simulink model "obs"  (R2014b)
settings: Solver=ode3  StartTime=0.0  StopTime=1875  FixedStep=0.5e-3  RelTol=1e-3
values from neighbouring files (symbols this model uses):
  C1_array = [10000 10000 20775.14128 59367.58362 2271.12322 25499.34704 24626.77363 22758.69305 1470.76099 16269.06063 343.94923 166277.12244 ... (44 elements, 11x4)]    [ecmparams_vsc.mat]    (also in load_sim_data.m = [ecmparams(1:3,2)'; ecmparams(4:6,2)'; ecmparams(7:9,2)']; load_sim_data_v2.m = [ecmparams(1:3,2)'; ecmparams(4:6,2)'; ecmparams(7:9,2)'])
  C2_array = [5000 5000 3386.51997 1284.26954 733.57385 21.9068258 408.44714 1025.29527 23.88432 4732.43934 4.98786 7213.94612 ... (44 elements, 11x4)]    [ecmparams_vsc.mat]    (also in load_sim_data.m = [ecmparams(1:3,4)'; ecmparams(4:6,4)'; ecmparams(7:9,4)']; load_sim_data_v2.m = [ecmparams(1:3,4)'; ecmparams(4:6,4)'; ecmparams(7:9,4)'])
  drive_profile = [0.003069801 0.003247245 0.003020715 0.003053892 0.002820143 0.003317081 0.003158873 0.002919445 0.002956375 0.002698265 0.002861501 0.002770798 ... (18750 elements, 1x18750)]    [drive_profile_ftp.mat]    (also in workspace.mat = [0 0 0 0 0 0 0 0 0 0 0 0 ... (521 elements, 1x521)]; workspace_2rc.mat; workspace_comparison.mat)
  drive_profile_index = [1 2 3 4 5 6 7 8 9 10 11 12 ... (18750 elements, 1x18750)]    [drive_profile_ftp.mat]    (also in load_sim_data_v2.m = drive_profile_index - 1; workspace.mat = [0 0.115384615385 0.230769230769 0.346153846154 0.4615384615; workspace_2rc.mat; workspace_comparison.mat)
  exp_vterm = [3.629339 3.628863 3.628776 3.628435 3.628006 3.627681 3.627586 3.627112 3.626967 3.626491 3.626216 3.625935 ... (18750 elements, 18750x1)]    [exp_vterm.mat]    (also in workspace_2rc.mat; workspace_comparison.mat)
  exp_vterm_index = [1 2 3 4 5 6 7 8 9 10 11 12 ... (18750 elements, 18750x1)]    [exp_vterm.mat]    (also in load_sim_data_v2.m = exp_vterm_index - 1)
  initial_soc = interp1(voc_soc_lut, voc_soc_lut_index, initial_vterm)    [load_sim_data.m]    (also in load_sim_data_v2.m)
  initial_temp = 25    [load_sim_data.m]    (also in load_sim_data_v2.m)
  initial_voc = interp1(voc_soc_lut_index, voc_soc_lut, initial_soc)    [load_sim_data.m]    (also in load_sim_data_v2.m)
  Q_total = 236.8    [load_sim_data.m]    (also in load_sim_data_v2.m = 350; workspace.mat = 44; workspace_2rc.mat = 44; workspace_comparison.mat = 44)
  R1 = interp2(temp_array, voc_array, R1_array, initial_temp, initial_voc)    [load_sim_data.m]    (also in load_sim_data_v2.m; workspace.mat = 0.00033425; workspace_2rc.mat = 0.0001483; workspace_comparison.mat = 0.0001483)
  R1_array = [0.001 0.001 0.00171 0.00621 0.00621 0.00495 0.00657 0.00419 0.01404 0.0095 0.00356 0.01783 ... (44 elements, 11x4)]    [ecmparams_vsc.mat]    (also in load_sim_data.m = [ecmparams(1:3,3)'; ecmparams(4:6,3)'; ecmparams(7:9,3)']; load_sim_data_v2.m = [ecmparams(1:3,3)'; ecmparams(4:6,3)'; ecmparams(7:9,3)'])
  R2 = interp2(temp_array, voc_array, R2_array, initial_temp, initial_voc)    [load_sim_data.m]    (also in load_sim_data_v2.m; workspace.mat = 0.000915125; workspace_2rc.mat = 0.0001594; workspace_comparison.mat = 0.0001594)
  R2_array = [0.001 0.001 0.00067 0.01044 0.00794 0.01181 0.0098 0.00694 0.00323 0.00236 0.02009 0.00195 ... (44 elements, 11x4)]    [ecmparams_vsc.mat]    (also in load_sim_data.m = [ecmparams(1:3,5)'; ecmparams(4:6,5)'; ecmparams(7:9,5)']; load_sim_data_v2.m = [ecmparams(1:3,5)'; ecmparams(4:6,5)'; ecmparams(7:9,5)'])
  Ri = interp2(temp_array, voc_array, Ri_array, initial_temp, initial_voc)    [load_sim_data.m]    (also in load_sim_data_v2.m; workspace.mat = 0.000736040625; workspace_2rc.mat = 0.0007932; workspace_comparison.mat = 0.0007932)
  Ri_array = [0.001 0.001 0.00089 0.02157 0.01286 0.00303 0.0054 0.0079 0.00204 0.01221 0.00632 0.00315 ... (44 elements, 11x4)]    [ecmparams_vsc.mat]    (also in load_sim_data.m = [ecmparams(1:3,1)'; ecmparams(4:6,1)'; ecmparams(7:9,1)']; load_sim_data_v2.m = [ecmparams(1:3,1)'; ecmparams(4:6,1)'; ecmparams(7:9,1)'])
  T_est = 0.02    [load_sim_data.m]    (also in load_sim_data_v2.m)
  temp_array = [15 25 35]    [load_sim_data.m]    (also in load_sim_data_v2.m)
  voc_array = [3 3.6 4.2]    [load_sim_data.m]    (also in load_sim_data_v2.m)
  voc_soc_lut = [3.07420931 3.44278771 3.51037487 3.58546258 3.63776945 3.68066188 3.73931818 3.84140797 3.94332291 4.0535654 4.18301283]    [emf_curve_single.mat]    (also in workspace.mat = [2.9985 3.0047 3.1504 3.2397 3.3026 3.3438 3.3699 3.3878 3.4; workspace_2rc.mat = [2.9985 3.0047 3.1504 3.2397 3.3026 3.3438 3.3699 3.3878 3.4; workspace_comparison.mat = [2.9985 3.0047 3.1504 3.2397 3.3026 3.3438 3.3699 3.3878 3.4)
  voc_soc_lut_index = [0 10 20 30 40 50 60 70 80 90 100]    [emf_curve_single.mat]    (also in workspace.mat = [0 1.6393442623 3.27868852459 4.91803278689 6.55737704918 8.; workspace_2rc.mat = [0 1.6393442623 3.27868852459 4.91803278689 6.55737704918 8.; workspace_comparison.mat = [0 1.6393442623 3.27868852459 4.91803278689 6.55737704918 8.)
libraries: fl_lib x16, nesl_utility x10
settings Model: Creator=OTG00077  LastModifiedBy=OTG00077
settings DebuggingCC: MultiTaskRateTransMsg=warning

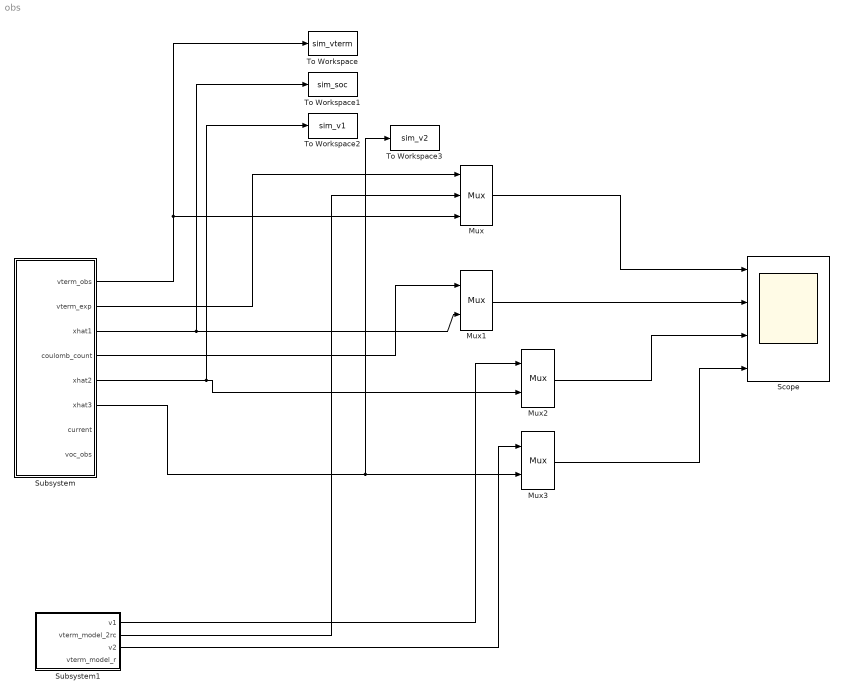
== system obs ==
  Mux : Mux  Inputs=3
  Mux1 : Mux  Inputs=2
  Mux2 : Mux  Inputs=2
  Mux3 : Mux  Inputs=2
  Scope : Scope  NumInputPorts=4
      settings: TimeRange=1875  YMin=3.458604651162791~0~-0.05~-0.05  YMax=3.741395348837209~40~0.009999999999999995~0.009999999999999995
  Subsystem : Subsystem
  Subsystem1 : Subsystem
  To Workspace : ToWorkspace  VariableName=sim_vterm  SampleTime=1
  To Workspace1 : ToWorkspace  VariableName=sim_soc  SampleTime=1
  To Workspace2 : ToWorkspace  VariableName=sim_v1  SampleTime=1
  To Workspace3 : ToWorkspace  VariableName=sim_v2  SampleTime=1
  wires:
  Subsystem/2(vterm_exp) -> Mux/1
  Subsystem1/2(vterm_model_2rc) -> Mux/2
  Subsystem/1(vterm_obs) -> To Workspace/1, Mux/3
  Subsystem/4(coulomb_count) -> Mux1/1
  Subsystem/3(xhat1) -> To Workspace1/1, Mux1/2
  Subsystem1/1(v1) -> Mux2/1
  Subsystem/5(xhat2) -> To Workspace2/1, Mux2/2
  Subsystem1/3(v2) -> Mux3/1
  Subsystem/6(xhat3) -> To Workspace3/1, Mux3/2
  Mux/1 -> Scope/1
  Mux1/1 -> Scope/2
  Mux2/1 -> Scope/3
  Mux3/1 -> Scope/4

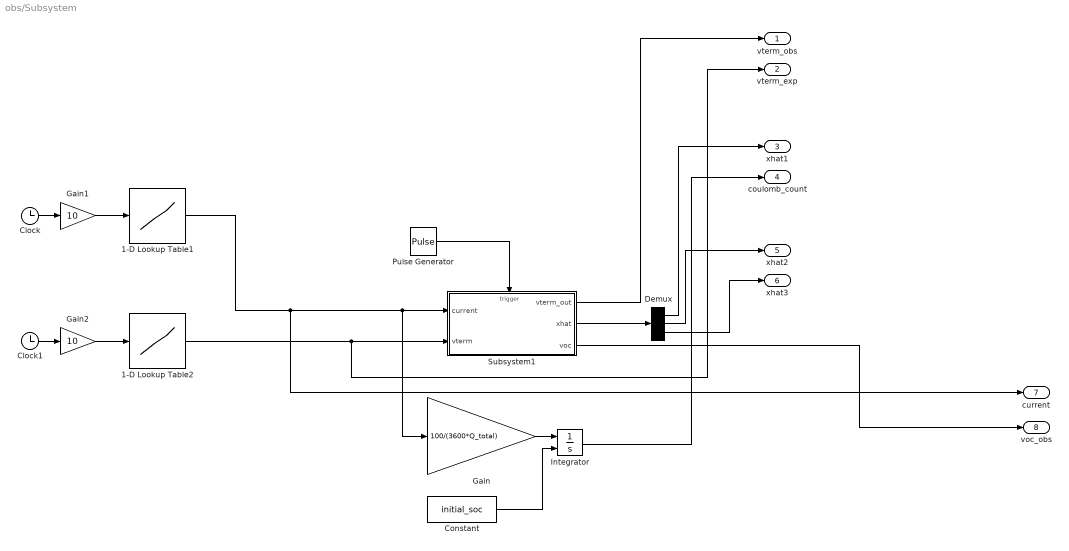
== system obs/Subsystem ==
  1-D Lookup Table1 : Lookup_n-D  NumberOfTableDimensions=1  BreakpointsForDimension1=drive_profile_index  Table=drive_profile  InternalRulePriority=Speed  RndMeth=Simplest  InputSameDT=on
  1-D Lookup Table2 : Lookup_n-D  NumberOfTableDimensions=1  BreakpointsForDimension1=exp_vterm_index  Table=exp_vterm  InternalRulePriority=Speed  RndMeth=Simplest  InputSameDT=on
  Clock : Clock
      settings: Decimation=100
  Clock1 : Clock
      settings: Decimation=100
  Constant : Constant  Value=initial_soc
  Demux : Demux  Outputs=3
  Gain : Gain  Gain=100/(3600*Q_total)
  Gain1 : Gain  Gain=10
  Gain2 : Gain  Gain=10
  Integrator : Integrator  InitialConditionSource=external  InitialCondition=initial_soc
  Pulse Generator : DiscretePulseGenerator  SampleTime=T_est/2
  Subsystem1 : Subsystem
  vterm_obs : Outport
  vterm_exp : Outport  Port=2
  xhat1 : Outport  Port=3
  coulomb_count : Outport  Port=4
  xhat2 : Outport  Port=5
  xhat3 : Outport  Port=6
  current : Outport  Port=7
  voc_obs : Outport  Port=8
  wires:
  Integrator/1 -> coulomb_count/1
  Gain/1 -> Integrator/1
  Pulse Generator/1 -> Subsystem1/Trigger
  1-D Lookup Table2/1 -> vterm_exp/1, Subsystem1/2(vterm)
  Subsystem1/2(xhat) -> Demux/1
  Clock1/1 -> Gain2/1
  Gain1/1 -> 1-D Lookup Table1/1
  Clock/1 -> Gain1/1
  1-D Lookup Table1/1 -> current/1, Gain/1, Subsystem1/1(current)
  Gain2/1 -> 1-D Lookup Table2/1
  Subsystem1/1(vterm_out) -> vterm_obs/1
  Demux/1 -> xhat1/1
  Constant/1 -> Integrator/2
  Demux/2 -> xhat2/1
  Demux/3 -> xhat3/1
  Subsystem1/3(voc) -> voc_obs/1

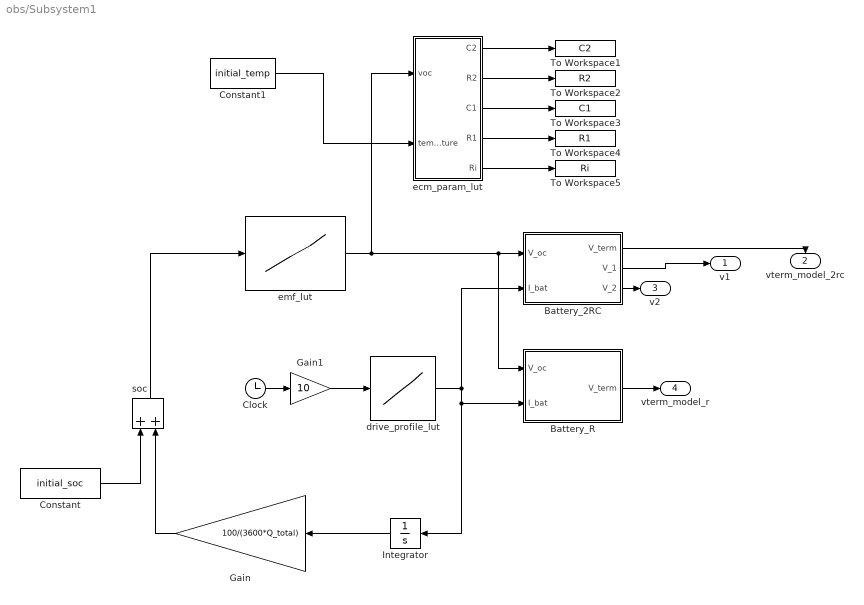
== system obs/Subsystem1 ==
  Battery_2RC : Subsystem
  Battery_R : Subsystem
  Clock : Clock
      settings: Decimation=100
  Constant : Constant  Value=initial_soc
  Constant1 : Constant  Value=initial_temp
  Gain : Gain  Gain=100/(3600*Q_total)
  Gain1 : Gain  Gain=10
  Integrator : Integrator
  To Workspace1 : ToWorkspace  VariableName=C2  SampleTime=-1
      settings: MaxDataPoints=1  Decimation=100
  To Workspace2 : ToWorkspace  VariableName=R2  SampleTime=-1
      settings: MaxDataPoints=1  Decimation=100
  To Workspace3 : ToWorkspace  VariableName=C1  SampleTime=-1
      settings: MaxDataPoints=1  Decimation=100
  To Workspace4 : ToWorkspace  VariableName=R1  SampleTime=-1
      settings: MaxDataPoints=1  Decimation=100
  To Workspace5 : ToWorkspace  VariableName=Ri  SampleTime=-1
      settings: MaxDataPoints=1  Decimation=100
  drive_profile_lut : Lookup_n-D  NumberOfTableDimensions=1  BreakpointsForDimension1=drive_profile_index  Table=drive_profile  InternalRulePriority=Speed  RndMeth=Simplest  InputSameDT=on
  "ecm_param_lut " : Subsystem
  emf_lut : Lookup_n-D  NumberOfTableDimensions=1  BreakpointsForDimension1=voc_soc_lut_index  Table=voc_soc_lut  InternalRulePriority=Speed  RndMeth=Simplest  InputSameDT=on
  soc : Sum
  v1 : Outport
  vterm_model_2rc : Outport  Port=2
  v2 : Outport  Port=3
  vterm_model_r : Outport  Port=4
  wires:
  "ecm_param_lut "/3(C1) -> To Workspace3/1
  "ecm_param_lut "/4(R1) -> To Workspace4/1
  Integrator/1 -> Gain/1
  Battery_2RC/2(V_1) -> v1/1
  Battery_2RC/3(V_2) -> v2/1
  Battery_2RC/1(V_term) -> vterm_model_2rc/1
  "ecm_param_lut "/5(Ri) -> To Workspace5/1
  Gain1/1 -> drive_profile_lut/1
  Battery_R/1(V_term) -> vterm_model_r/1
  "ecm_param_lut "/1(C2) -> To Workspace1/1
  "ecm_param_lut "/2(R2) -> To Workspace2/1
  drive_profile_lut/1 -> Battery_R/2(I_bat), Integrator/1, Battery_2RC/2(I_bat)
  Clock/1 -> Gain1/1
  emf_lut/1 -> "ecm_param_lut "/1(voc), Battery_R/1(V_oc), Battery_2RC/1(V_oc)
  Constant/1 -> soc/1
  Gain/1 -> soc/2
  soc/1 -> emf_lut/1
  Constant1/1 -> "ecm_param_lut "/2(temperature)

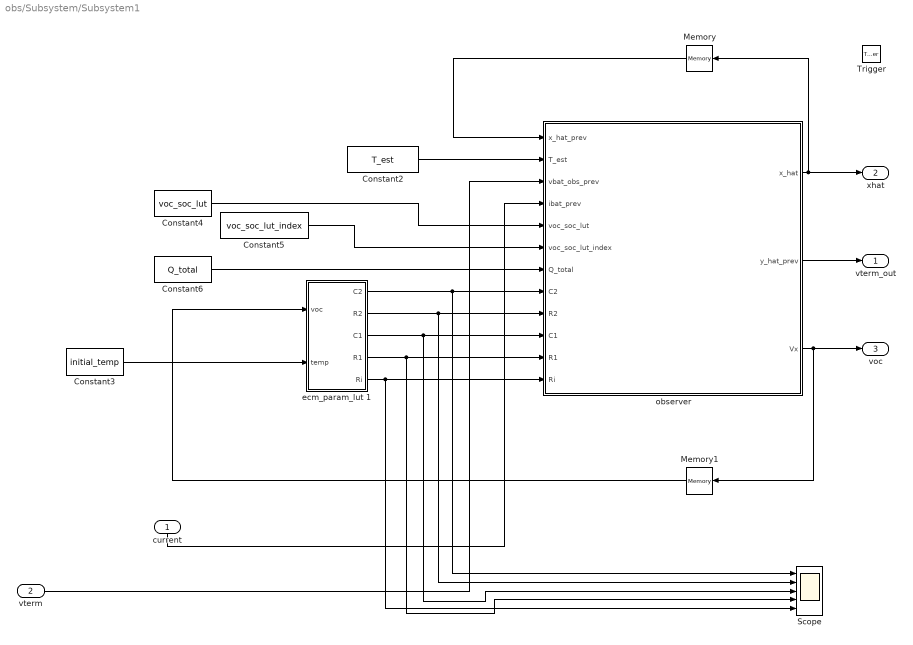
== system obs/Subsystem/Subsystem1 ==
  current : Inport
  vterm : Inport  Port=2
  Trigger : TriggerPort  PortDimensions=1
  Constant2 : Constant  Value=T_est
  Constant3 : Constant  Value=initial_temp
  Constant4 : Constant  Value=voc_soc_lut
  Constant5 : Constant  Value=voc_soc_lut_index
  Constant6 : Constant  Value=Q_total
  Memory : Memory  X0=[initial_soc; 0; 0]  InheritSampleTime=on  LinearizeMemory=on  LinearizeAsDelay=on
  Memory1 : Memory  X0=initial_voc  InheritSampleTime=on  LinearizeMemory=on  LinearizeAsDelay=on
  Scope : Scope  NumInputPorts=5
      settings: TimeRange=1875  YMin=22~0.0001697~250~0.0001672~0.0008025  YMax=22.8~0.0001701~265~0.000168~0.000803
  ecm_param_lut 1 : Subsystem
  observer : MATLAB Function  TreatAsAtomicUnit=on
  vterm_out : Outport
  xhat : Outport  Port=2
  voc : Outport  Port=3
  wires:
  observer/3(Vx) -> voc/1, Memory1/1
  Memory/1 -> observer/1(x_hat_prev)
  Memory1/1 -> ecm_param_lut 1/1(voc)
  Constant6/1 -> observer/7(Q_total)
  Constant5/1 -> observer/6(voc_soc_lut_index)
  ecm_param_lut 1/5(Ri) -> Scope/5, observer/12(Ri)
  observer/1(x_hat) -> xhat/1, Memory/1
  Constant2/1 -> observer/2(T_est)
  Constant4/1 -> observer/5(voc_soc_lut)
  ecm_param_lut 1/3(C1) -> Scope/3, observer/10(C1)
  ecm_param_lut 1/1(C2) -> Scope/1, observer/8(C2)
  ecm_param_lut 1/4(R1) -> Scope/4, observer/11(R1)
  ecm_param_lut 1/2(R2) -> Scope/2, observer/9(R2)
  vterm/1 -> observer/3(vbat_obs_prev)
  observer/2(y_hat_prev) -> vterm_out/1
  current/1 -> observer/4(ibat_prev)
  Constant3/1 -> ecm_param_lut 1/2(temp)

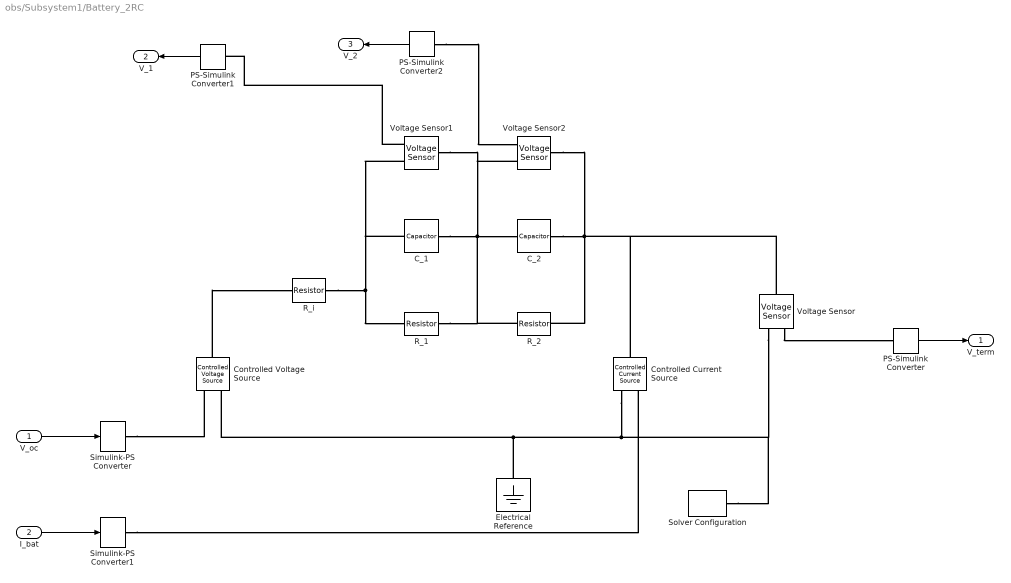
== system obs/Subsystem1/Battery_2RC ==
  V_oc : Inport
  I_bat : Inport  Port=2
  C_1 : fl_lib/Electrical/Electrical Elements/Capacitor  c=C1 F  r=0 Ohm  g=0 1/Ohm  i_specify=off  i_priority=High  i=0 A  v_specify=off  v_priority=High  v=0 V  vc_specify=off  vc_priority=High  vc=0 V
  C_2 : fl_lib/Electrical/Electrical Elements/Capacitor  c=C2 F  r=0 Ohm  g=0 1/Ohm  i_specify=off  i_priority=High  i=0 A  v_specify=off  v_priority=High  v=0 V  vc_specify=off  vc_priority=High  vc=0 V
  Controlled Current Source : fl_lib/Electrical/Electrical Sources/Controlled Current Source
  Controlled Voltage Source : fl_lib/Electrical/Electrical Sources/Controlled Voltage Source
  Electrical Reference : fl_lib/Electrical/Electrical Elements/Electrical Reference
  PS-Simulink Converter : nesl_utility/PS-Simulink Converter  PhysicalDomain=network_engine_domain  SubClassName=ps_output  LeftPortType=input  RightPortType=output  PseudoPeriodic=off  Frequencies=[]  Unit=1  AffineConversion=off
  PS-Simulink Converter1 : nesl_utility/PS-Simulink Converter  PhysicalDomain=network_engine_domain  SubClassName=ps_output  LeftPortType=input  RightPortType=output  PseudoPeriodic=off  Frequencies=[]  Unit=1  AffineConversion=off
  PS-Simulink Converter2 : nesl_utility/PS-Simulink Converter  PhysicalDomain=network_engine_domain  SubClassName=ps_output  LeftPortType=input  RightPortType=output  PseudoPeriodic=off  Frequencies=[]  Unit=1  AffineConversion=off
  R_1 : fl_lib/Electrical/Electrical Elements/Resistor  R=R1 Ohm  i_specify=off  i_priority=High  i=0 A  v_specify=off  v_priority=High  v=0 V
  R_2 : fl_lib/Electrical/Electrical Elements/Resistor  R=R2 Ohm  i_specify=off  i_priority=High  i=0 A  v_specify=off  v_priority=High  v=0 V
  R_i : fl_lib/Electrical/Electrical Elements/Resistor  R=Ri Ohm  i_specify=off  i_priority=High  i=0 A  v_specify=off  v_priority=High  v=0 V
  Simulink-PS Converter : nesl_utility/Simulink-PS Converter  PhysicalDomain=network_engine_domain  SubClassName=ps_input  LeftPortType=input  RightPortType=output  PseudoPeriodic=off  Frequencies=[]  NoiseDistribution=none  NoiseParameters=[]  Unit=1  AffineConversion=off  InputFiltering=off  SimscapeFilterOrder=1  InputFilterTimeConstant=0.001  UdotUserProvided=1
  Simulink-PS Converter1 : nesl_utility/Simulink-PS Converter  PhysicalDomain=network_engine_domain  SubClassName=ps_input  LeftPortType=input  RightPortType=output  PseudoPeriodic=off  Frequencies=[]  NoiseDistribution=none  NoiseParameters=[]  Unit=1  AffineConversion=off  InputFiltering=off  SimscapeFilterOrder=1  InputFilterTimeConstant=0.001  UdotUserProvided=1
  Solver Configuration : nesl_utility/Solver Configuration  PhysicalDomain=network_engine_domain  SubClassName=solver  LeftPortType=input  RightPortType=generic  Accelerate=off  Tones=[]  Harmonics=[]  SimulateNoise=off  Profile=off  UseLocalSampling=off  EnableSwitchedLinearOptims=on  FrequencyDomain=off  UseCCode=off  RelTol=0.001  AbsTol=1e-06  MinStep=1e-09  ToWorkspace=off  DoDC=off  ResidualTolerance=1e-09  UseLocalSolver=off  LocalSolverChoice=NE_BACKWARD_EULER_ADVANCER  LocalSolverSampleTime=0.001  DoFixedCost=off  MaxNonlinIter=3  MaxModeIter=2  LinearAlgebra=Sparse  DelaysMemoryBudget=1024  AutomaticFiltering=on  FilteringTimeConstant=0.001
  Voltage Sensor : fl_lib/Electrical/Electrical Sensors/Voltage Sensor
  Voltage Sensor1 : fl_lib/Electrical/Electrical Sensors/Voltage Sensor
  Voltage Sensor2 : fl_lib/Electrical/Electrical Sensors/Voltage Sensor
  V_term : Outport
  V_1 : Outport  Port=2
  V_2 : Outport  Port=3
  wires:
  V_oc/1 -> Simulink-PS Converter/1
  PS-Simulink Converter/1 -> V_term/1
  I_bat/1 -> Simulink-PS Converter1/1
  PS-Simulink Converter1/1 -> V_1/1
  PS-Simulink Converter2/1 -> V_2/1
  connections:
  R_i/RConn1 -- Voltage Sensor1/RConn2 -- C_1/LConn1 -- R_1/LConn1
  C_1/RConn1 -- Voltage Sensor2/RConn2 -- Voltage Sensor1/LConn1 -- R_2/LConn1 -- R_1/RConn1 -- C_2/LConn1
  C_2/RConn1 -- Voltage Sensor2/LConn1 -- R_2/RConn1 -- Controlled Current Source/LConn1 -- Voltage Sensor/LConn1
  Controlled Voltage Source/LConn1 -- R_i/LConn1
  Simulink-PS Converter/RConn1 -- Controlled Voltage Source/RConn1
  Voltage Sensor/RConn1 -- PS-Simulink Converter/LConn1
  Controlled Current Source/RConn2 -- Solver Configuration/RConn1 -- Voltage Sensor/RConn2 -- Electrical Reference/LConn1 -- Controlled Voltage Source/RConn2
  Simulink-PS Converter1/RConn1 -- Controlled Current Source/RConn1
  Voltage Sensor1/RConn1 -- PS-Simulink Converter1/LConn1
  PS-Simulink Converter2/LConn1 -- Voltage Sensor2/RConn1

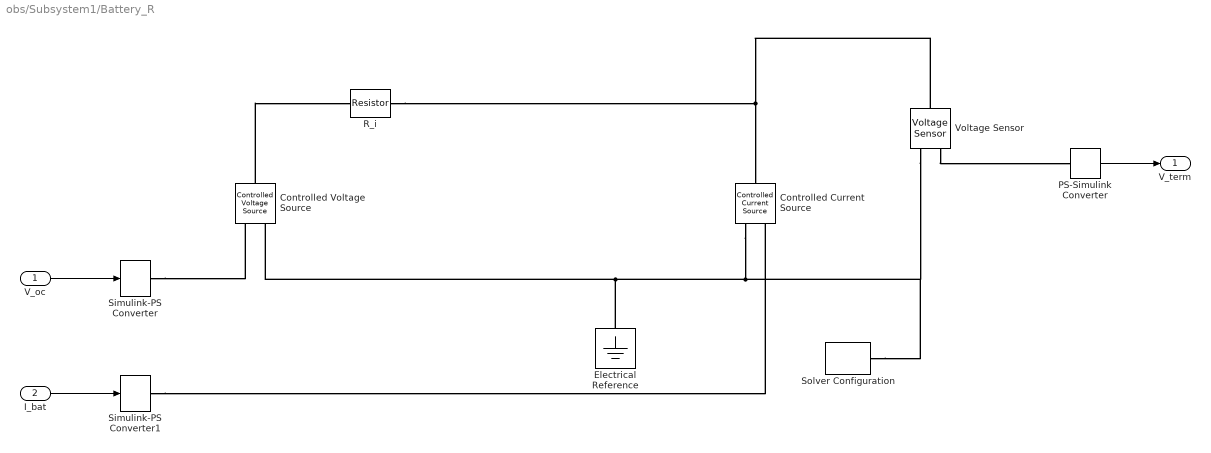
== system obs/Subsystem1/Battery_R ==
  V_oc : Inport
  I_bat : Inport  Port=2
  Controlled Current Source : fl_lib/Electrical/Electrical Sources/Controlled Current Source
  Controlled Voltage Source : fl_lib/Electrical/Electrical Sources/Controlled Voltage Source
  Electrical Reference : fl_lib/Electrical/Electrical Elements/Electrical Reference
  PS-Simulink Converter : nesl_utility/PS-Simulink Converter  PhysicalDomain=network_engine_domain  SubClassName=ps_output  LeftPortType=input  RightPortType=output  PseudoPeriodic=off  Frequencies=[]  Unit=1  AffineConversion=off
  R_i : fl_lib/Electrical/Electrical Elements/Resistor  R=Ri+R1+R2 Ohm  i_specify=off  i_priority=High  i=0 A  v_specify=off  v_priority=High  v=0 V
  Simulink-PS Converter : nesl_utility/Simulink-PS Converter  PhysicalDomain=network_engine_domain  SubClassName=ps_input  LeftPortType=input  RightPortType=output  PseudoPeriodic=off  Frequencies=[]  NoiseDistribution=none  NoiseParameters=[]  Unit=1  AffineConversion=off  InputFiltering=off  SimscapeFilterOrder=1  InputFilterTimeConstant=0.001  UdotUserProvided=1
  Simulink-PS Converter1 : nesl_utility/Simulink-PS Converter  PhysicalDomain=network_engine_domain  SubClassName=ps_input  LeftPortType=input  RightPortType=output  PseudoPeriodic=off  Frequencies=[]  NoiseDistribution=none  NoiseParameters=[]  Unit=1  AffineConversion=off  InputFiltering=off  SimscapeFilterOrder=1  InputFilterTimeConstant=0.001  UdotUserProvided=1
  Solver Configuration : nesl_utility/Solver Configuration  PhysicalDomain=network_engine_domain  SubClassName=solver  LeftPortType=input  RightPortType=generic  Accelerate=off  Tones=[]  Harmonics=[]  SimulateNoise=off  Profile=off  UseLocalSampling=off  EnableSwitchedLinearOptims=on  FrequencyDomain=off  UseCCode=off  RelTol=0.001  AbsTol=1e-06  MinStep=1e-09  ToWorkspace=off  DoDC=off  ResidualTolerance=1e-09  UseLocalSolver=off  LocalSolverChoice=NE_BACKWARD_EULER_ADVANCER  LocalSolverSampleTime=0.001  DoFixedCost=off  MaxNonlinIter=3  MaxModeIter=2  LinearAlgebra=Sparse  DelaysMemoryBudget=1024  AutomaticFiltering=on  FilteringTimeConstant=0.001
  Voltage Sensor : fl_lib/Electrical/Electrical Sensors/Voltage Sensor
  V_term : Outport
  wires:
  V_oc/1 -> Simulink-PS Converter/1
  PS-Simulink Converter/1 -> V_term/1
  I_bat/1 -> Simulink-PS Converter1/1
  connections:
  Voltage Sensor/LConn1 -- Controlled Current Source/LConn1 -- R_i/RConn1
  Controlled Voltage Source/LConn1 -- R_i/LConn1
  Simulink-PS Converter/RConn1 -- Controlled Voltage Source/RConn1
  Voltage Sensor/RConn1 -- PS-Simulink Converter/LConn1
  Controlled Current Source/RConn2 -- Solver Configuration/RConn1 -- Voltage Sensor/RConn2 -- Electrical Reference/LConn1 -- Controlled Voltage Source/RConn2
  Simulink-PS Converter1/RConn1 -- Controlled Current Source/RConn1

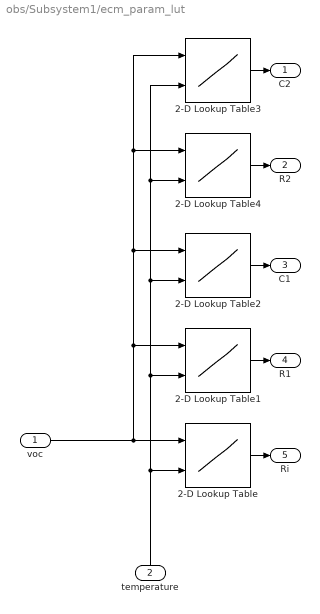
== system obs/Subsystem1/ecm_param_lut  ==
  voc : Inport
  temperature : Inport  Port=2
  2-D Lookup Table : Lookup_n-D  BreakpointsForDimension1=voc_array  BreakpointsForDimension2=temp_array  Table=Ri_array  InternalRulePriority=Speed  RndMeth=Simplest  InputSameDT=on
  2-D Lookup Table1 : Lookup_n-D  BreakpointsForDimension1=voc_array  BreakpointsForDimension2=temp_array  Table=R1_array  InternalRulePriority=Speed  RndMeth=Simplest  InputSameDT=on
  2-D Lookup Table2 : Lookup_n-D  BreakpointsForDimension1=voc_array  BreakpointsForDimension2=temp_array  Table=C1_array  InternalRulePriority=Speed  RndMeth=Simplest  InputSameDT=on
  2-D Lookup Table3 : Lookup_n-D  BreakpointsForDimension1=voc_array  BreakpointsForDimension2=temp_array  Table=C2_array  InternalRulePriority=Speed  RndMeth=Simplest  InputSameDT=on
  2-D Lookup Table4 : Lookup_n-D  BreakpointsForDimension1=voc_array  BreakpointsForDimension2=temp_array  Table=R2_array  InternalRulePriority=Speed  RndMeth=Simplest  InputSameDT=on
  C2 : Outport
  R2 : Outport  Port=2
  C1 : Outport  Port=3
  R1 : Outport  Port=4
  Ri : Outport  Port=5
  wires:
  voc/1 -> 2-D Lookup Table1/1, 2-D Lookup Table2/1, 2-D Lookup Table4/1, 2-D Lookup Table3/1, 2-D Lookup Table/1
  2-D Lookup Table2/1 -> C1/1
  2-D Lookup Table4/1 -> R2/1
  2-D Lookup Table/1 -> Ri/1
  2-D Lookup Table1/1 -> R1/1
  2-D Lookup Table3/1 -> C2/1
  temperature/1 -> 2-D Lookup Table3/2, 2-D Lookup Table4/2, 2-D Lookup Table2/2, 2-D Lookup Table1/2, 2-D Lookup Table/2

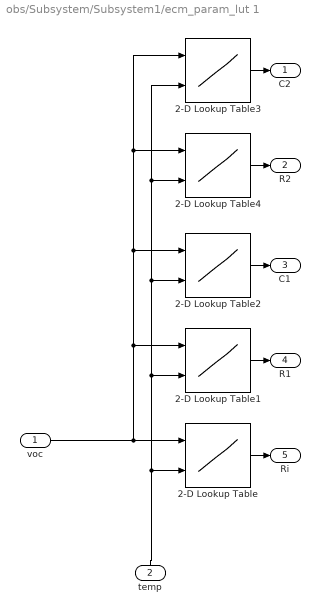
== system obs/Subsystem/Subsystem1/ecm_param_lut 1 ==
  voc : Inport
  temp : Inport  Port=2
  2-D Lookup Table : Lookup_n-D  BreakpointsForDimension1=voc_array  BreakpointsForDimension2=temp_array  BeginIndexSearchUsingPreviousIndexResult=on  Table=Ri_array  ExtrapMethod=Clip  DiagnosticForOutOfRangeInput=Warning  UseLastTableValue=on  InternalRulePriority=Speed  RndMeth=Simplest  InputSameDT=on
  2-D Lookup Table1 : Lookup_n-D  BreakpointsForDimension1=voc_array  BreakpointsForDimension2=temp_array  BeginIndexSearchUsingPreviousIndexResult=on  Table=R1_array  ExtrapMethod=Clip  UseLastTableValue=on  InternalRulePriority=Speed  RndMeth=Simplest  InputSameDT=on
  2-D Lookup Table2 : Lookup_n-D  BreakpointsForDimension1=voc_array  BreakpointsForDimension2=temp_array  BeginIndexSearchUsingPreviousIndexResult=on  Table=C1_array  ExtrapMethod=Clip  UseLastTableValue=on  InternalRulePriority=Speed  RndMeth=Simplest  InputSameDT=on
  2-D Lookup Table3 : Lookup_n-D  BreakpointsForDimension1=voc_array  BreakpointsForDimension2=temp_array  BeginIndexSearchUsingPreviousIndexResult=on  Table=C2_array  ExtrapMethod=Clip  DiagnosticForOutOfRangeInput=Warning  UseLastTableValue=on  InternalRulePriority=Speed  RndMeth=Simplest  InputSameDT=on
  2-D Lookup Table4 : Lookup_n-D  BreakpointsForDimension1=voc_array  BreakpointsForDimension2=temp_array  BeginIndexSearchUsingPreviousIndexResult=on  Table=R2_array  ExtrapMethod=Clip  UseLastTableValue=on  InternalRulePriority=Speed  RndMeth=Simplest  InputSameDT=on
  C2 : Outport
  R2 : Outport  Port=2
  C1 : Outport  Port=3
  R1 : Outport  Port=4
  Ri : Outport  Port=5
  wires:
  voc/1 -> 2-D Lookup Table1/1, 2-D Lookup Table2/1, 2-D Lookup Table4/1, 2-D Lookup Table3/1, 2-D Lookup Table/1
  2-D Lookup Table2/1 -> C1/1
  2-D Lookup Table4/1 -> R2/1
  2-D Lookup Table/1 -> Ri/1
  2-D Lookup Table1/1 -> R1/1
  2-D Lookup Table3/1 -> C2/1
  temp/1 -> 2-D Lookup Table3/2, 2-D Lookup Table4/2, 2-D Lookup Table2/2, 2-D Lookup Table1/2, 2-D Lookup Table/2

== matlab function obs/Subsystem/Subsystem1/observer ==
  data: x_hat_prev input size=[3,1]; x_hat output size=[3,1]; T_est input; vbat_obs_prev input; ibat_prev input; voc_soc_lut input; voc_soc_lut_index input; Q_total input; C2 input; R2 input; C1 input; R1 input; Ri input; y_hat_prev output; Vx output
function [x_hat,y_hat_prev,Vx] = obs(x_hat_prev, T_est, ...
    vbat_obs_prev, ibat_prev, voc_soc_lut, voc_soc_lut_index,Q_total, C2, R2, C1, R1, Ri)
%#codegen

%1s gain
L=[0.2; 0.2; 0.2];
%L=0;

%A matrix
A=eye(3);
A(2,2)=1-T_est/(R1*C1);
A(3,3)=1-T_est/(R2*C2);

%B matrix
B=[100*T_est/(3600*Q_total); T_est/C1; T_est/C2];

%calculate voc
Vx=interp1(voc_soc_lut_index,voc_soc_lut,x_hat_prev(1));

y_hat_prev=Vx+Ri*ibat_prev+x_hat_prev(2)+x_hat_prev(3);

%current state estimate
x_hat=A*x_hat_prev+B*ibat_prev+L*(vbat_obs_prev-y_hat_prev);
% A
% x_hat_prev
% B
% C
% L
